simulink model "rozniczkujacy"  (R2013a)
settings: Solver=ode45  StartTime=0.0  StopTime=10.0  MaxStep=0.01  RelTol=1e-3
values from neighbouring files (symbols this model uses):
  k = 3    [calkujacy.m]    (also in lab3.m = 1)
  T = 2    [calkujacy.m]    (also in lab3.m)
  x = 5    [lab3.m]
settings Model: Creator=L13-3  LastModifiedBy=Junior
settings DataIOCC: SignalLoggingSaveFormat=ModelDataLogs
settings DebuggingCC: UnderspecifiedInitializationDetection=Simplified  MultiTaskDSMMsg=warning  MultiTaskCondExecSysMsg=none  StateNameClashWarn=none  StrictBusMsg=ErrorOnBusTreatedAsVector
settings RTWCC: IncludeERTFirstTime=on
settings GRTTargetCC: CodeReplacementLibrary=None  CPPClassGenCompliant=on

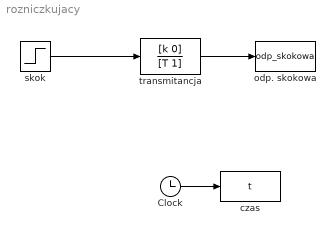
== system rozniczkujacy ==
  Clock : Clock
  czas : ToWorkspace  VariableName=t  SampleTime=-1
  odp. skokowa : ToWorkspace  VariableName=odp_skokowa  SampleTime=-1
  skok : Step  Time=x  SampleTime=0
  transmitancja : TransferFcn  Numerator=[k 0]  Denominator=[T 1]
  wires:
  skok/1 -> transmitancja/1
  Clock/1 -> czas/1
  transmitancja/1 -> odp. skokowa/1
